simulink library "CTRL_DSI_MomentMethod"  (R2023b)
settings: Solver=VariableStepAuto  StartTime=0.0  StopTime=10.0  RelTol=1e-3
settings Model: Creator=blatak  LastModifiedBy=blatak
settings ModelReferenceCC: EnableRefExpFcnMdlSchedulingChecks=on

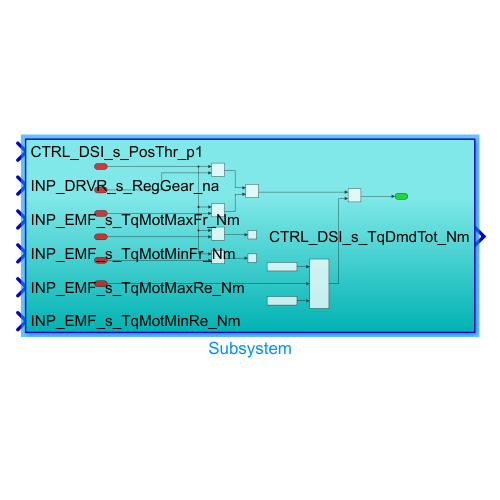
[thumbnail: Simulink's stored preview of the top-level diagram]
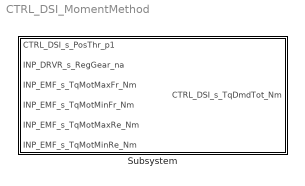
== system CTRL_DSI_MomentMethod ==
  Subsystem : Subsystem

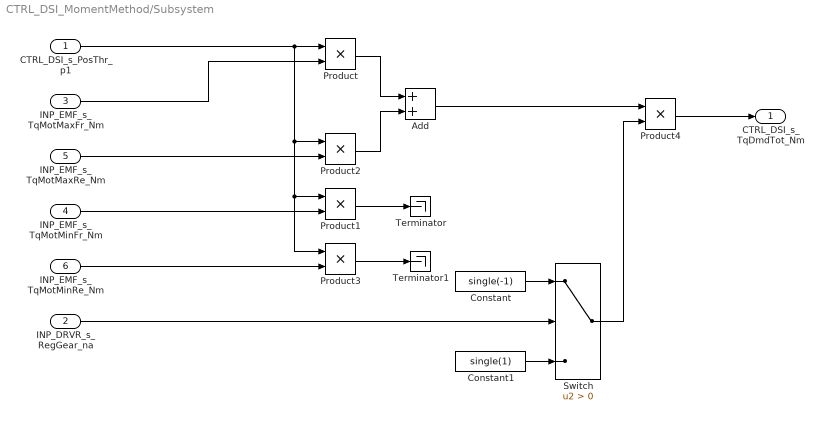
== system CTRL_DSI_MomentMethod/Subsystem ==
  CTRL_DSI_s_PosThr_p1 : Inport
  INP_DRVR_s_RegGear_na : Inport  Port=2
  INP_EMF_s_TqMotMaxFr_Nm : Inport  Port=3
  INP_EMF_s_TqMotMinFr_Nm : Inport  Port=4
  INP_EMF_s_TqMotMaxRe_Nm : Inport  Port=5
  INP_EMF_s_TqMotMinRe_Nm : Inport  Port=6
  Add : Sum
  Constant : Constant  Value=single(-1)
  Constant1 : Constant  Value=single(1)
  Product{,1..4} (5 alike) : Product
  Switch : Switch  Criteria=u2 > Threshold  SaturateOnIntegerOverflow=off  InputSameDT=off
  Terminator : Terminator
  Terminator1 : Terminator
  CTRL_DSI_s_TqDmdTot_Nm : Outport
  wires:
  INP_EMF_s_TqMotMinRe_Nm/1 -> Product3/2
  CTRL_DSI_s_PosThr_p1/1 -> Product3/1, Product1/1, Product2/1, Product/1
  Add/1 -> Product4/1
  INP_EMF_s_TqMotMaxFr_Nm/1 -> Product/2
  Constant/1 -> Switch/1
  Product4/1 -> CTRL_DSI_s_TqDmdTot_Nm/1
  Product/1 -> Add/1
  Product1/1 -> Terminator/1
  INP_EMF_s_TqMotMinFr_Nm/1 -> Product1/2
  Product3/1 -> Terminator1/1
  Product2/1 -> Add/2
  Switch/1 -> Product4/2
  INP_EMF_s_TqMotMaxRe_Nm/1 -> Product2/2
  INP_DRVR_s_RegGear_na/1 -> Switch/2
  Constant1/1 -> Switch/3
